simulink model "exDroopB_sim"  (R2014b)
settings: Solver=ode45  SolverMode=SingleTasking  StartTime=0.0  StopTime=15  MaxStep=0.0015  RelTol=1e-08
values from neighbouring files (symbols this model uses):
  bus1_vd = 2^0.5*1e3    (= 1414.21356237)    [ex3busPV.m]    (also in exLongLinePV.m = 141421.356237)
  Cbus_ext = 1e6*mpcC.bus(ssgen,BS)./(ws*baseV(ssgen).^2)    [exDroopA.m]    (also in exDroopB.m; exSyncGenPVinv.m)
  droop_Pref = 0.25*Pbase    (= 75000000)    [ex7busLongLine.m]    (also in exDroopA.m = mpc.gen(2:end,PG)*1e6; exDroopB.m = mpc.gen(:,PG)*1e6; exSyncGenPVinv.m = droop_Pref( [1:(synrp-1),(synrp+1):end]  ))
  droop_R = DROOP_R_GAIN_CNST./Prt    [ex7busLongLine.m]    (also in exDroopA.m; exDroopB.m)
  If_dc = 0.2*Prt./Ert    [ex14busSGandPV.m]    (also in ex7busLongLine.m = Prt./(60*Vf_dc); exDroopA.m = Prt./(60*Vf_dc); exDroopB.m = Prt./(60*Vf_dc); exSyncGenPVinv.m)
  J = J_GAIN_CNST*Prt/ws    [ex14busSGandPV.m]    (also in ex2busStability.m = 7.63943726841; ex7busLongLine.m = 2387.32414638; ex9busSG.m = J_GAIN_CNST*Pmax_gens/ws; exDroopA.m)
  Jtot = sum(J)    [exDroopB.m]
  Kd = KD_GAIN_CNST*J*ws    [ex14busSGandPV.m]    (also in ex2busStability.m = 24000; ex7busLongLine.m; ex9busSG.m; exDroopA.m)
  L0 = 0.1*Ld    [ex14busSGandPV.m]    (also in ex7busLongLine.m; exDroopA.m; exDroopB.m; exSyncGenPVinv.m)
  Laf = (2^0.5)*Ert./(ws*If_dc)    [ex14busSGandPV.m]    (also in ex7busLongLine.m; exDroopA.m; exDroopB.m; exSyncGenPVinv.m = (2^0.5)*5*Ert.^2./(ws*Prt))
  Lb2 = 2*Ld.*Lff - 3*Laf.^2    [ex14busSGandPV.m]    (also in ex7busLongLine.m; exDroopA.m; exDroopB.m; exSyncGenPVinv.m)
  Ld = 0.6*Lpu    [ex14busSGandPV.m]    (also in ex7busLongLine.m = 0.3*Lpu; exDroopA.m = 0.3*Lpu; exDroopB.m = 0.3*Lpu; exSyncGenPVinv.m)
  Lff = 2*Laf.^2./Ld    [ex14busSGandPV.m]    (also in ex7busLongLine.m; exDroopA.m; exDroopB.m; exSyncGenPVinv.m)
  Lq = Ld    [ex14busSGandPV.m]    (also in ex7busLongLine.m; exDroopA.m; exDroopB.m; exSyncGenPVinv.m)
  poles_2Jws = poles./(2*J*ws)    [ex14busSGandPV.m]    (also in ex2busStability.m = poles./(2*ws*J); ex7busLongLine.m; ex9busSG.m = poles./(2*ws*J); exDroopA.m)
  Ra = 0.05*Ert.^2./Prt    [ex14busSGandPV.m]    (also in ex7busLongLine.m = 0.01*Ert.^2./Prt; exDroopA.m = 0.01*Ert.^2./Prt; exDroopB.m = 0.01*Ert.^2./Prt; exSyncGenPVinv.m)
  Rf = Lff/1.2    [ex14busSGandPV.m]    (also in ex7busLongLine.m = Vf_dc./If_dc; exDroopA.m = Vf_dc./If_dc; exDroopB.m = Vf_dc./If_dc; exSyncGenPVinv.m)
  ssbus = [1; 2; 3; 6; 8]    [ex14busSGandPV.m]    (also in ex9busSG.m = [1 ; Genbus]; exDroopA.m = mpc.gen(:,GEN_BUS); exDroopB.m = mpc.gen(:,GEN_BUS); exLargeSysStability.m = mpc.gen(:,GEN_BUS))
  step_gen_num = 1    [exDroopB.m]
  step_size = 30e3    (= 30000)    [ex2busStability.m]    (also in exDroopB.m = 0)
  step_time = 9    [ex2busStability.m]    (also in ex3busPV.m = 0.05; exDroopB.m = 10; exLongLinePV.m = 1; syncMachVsSwing.m = 5)
  vcap_init_0 = 0*vppa    [exDroopA.m]    (also in exDroopB.m; exSyncGenPVinv.m)
  vcap_init_d = real(vppa)    [exDroopA.m]    (also in exDroopB.m; exSyncGenPVinv.m)
  vcap_init_q = imag(vppa)    [exDroopA.m]    (also in exDroopB.m; exSyncGenPVinv.m)
  Vf_dc = If_dc.*Rf    [ex14busSGandPV.m]    (also in ex7busLongLine.m = 500 * ones(size(Ert)); exDroopA.m = 500 * ones(size(Ert)); exDroopB.m = 500 * ones(size(Ert)); exSyncGenPVinv.m)
  ws = 2*pi*50    (= 314.159265359)    [ex14busSGandPV.m]    (also in ex2busStability.m; ex3busPV.m; ex7busLongLine.m; ex9busSG.m)
undefined symbols (not defined in the file or in its folder): Anet, Bnet, Cnet, Dnet, full
settings Model: Creator=COPEC  LastModifiedBy=Juri
settings OptimizationCC: BlockReduction=off  BooleanDataType=off
settings DebuggingCC: SaveWithParameterizedLinksMsg=none  UnderspecifiedInitializationDetection=Classic  MergeDetectMultiDrivingBlocksExec=none  SignalResolutionControl=TryResolveAllWithWarning  SolverPrmCheckMsg=none  FrameProcessingCompatibilityMsg=error
settings HardwareCC: TargetUnknown=on

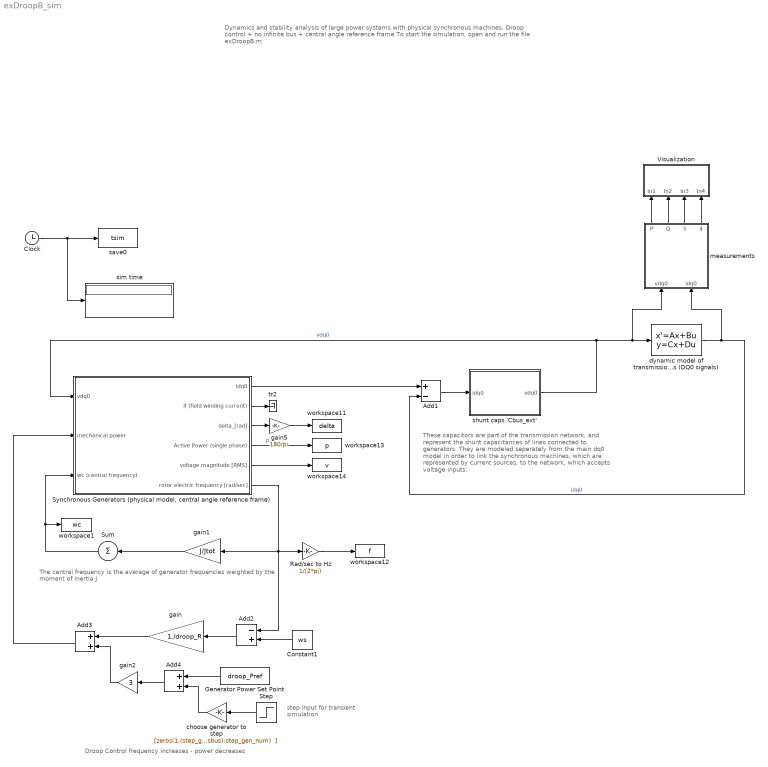
== system exDroopB_sim ==
  note: step input
      | for transient simulation
  note: Droop Control
      | frequency increases - power decreases
  note: Dynamics and stability analysis of large power systems
      | with physical synchronous machines.
      | Droop control + no infinite bus + central angle reference frame
      |
      | To start the simulation, open and run the file
      | exDroopB.m
  note: These capacitors are part of the transmission network, and represent the shunt capacitances of lines connected to generators. They are modeled seperately from the main dq0 model in order to link the synchronous machines, which are represented by current sources, to the network, which accepts voltage inputs.
  note: The central frequency is the average of generator
      | frequencies weighted by the moment of inertia J
  Add1 : Sum  Inputs=+-
  Add2 : Sum  Inputs=-+
  Add3 : Sum
  Add4 : Sum
  Clock : Clock
  Constant1 : Constant  Value=ws
  Generator Power Set Point : Constant  Value=droop_Pref
  Rad/sec to Hz : Gain  Gain=1/(2*pi)
  Step : Step  Time=step_time  After=step_size  SampleTime=0
  Sum : Sum  Inputs=+
  "Synchronous Generators (physical model, central angle reference frame)" : Subsystem
  Visualization : Subsystem
  choose generator to step : Gain  Gain="[zeros(1,(step_gen_num-1)) , 1 ,  zeros(1,length(ssbus)-step_gen_num)  ]"
  dynamic model of transmission network with integrated loads (DQ0 signals) : StateSpace  A=full(Anet)  B=full(Bnet)  C=full(Cnet)  D=full(Dnet)  X0=0
  gain : Gain  Gain=1./droop_R
  gain1 : Gain  Gain=J/Jtot
  gain2 : Gain  Gain=3
  gain5 : Gain  Gain=180/pi
  measurements : Subsystem
  save0 : ToWorkspace  VariableName=tsim  SampleTime=-1
  "shunt caps 'Cbus_ext' " : Subsystem
  sim time : Display
  tr2 : Terminator
  workspace1 : ToWorkspace  VariableName=wc  SampleTime=-1
  workspace11 : ToWorkspace  VariableName=delta  SampleTime=-1
  workspace12 : ToWorkspace  VariableName=f  SampleTime=-1
  workspace13 : ToWorkspace  VariableName=p  SampleTime=-1
  workspace14 : ToWorkspace  VariableName=v  SampleTime=-1
  wires:
  Clock/1 -> sim time/1, save0/1
  "Synchronous Generators (physical model, central angle reference frame)"/2(if (field winding current)) -> tr2/1
  "Synchronous Generators (physical model, central angle reference frame)"/3(delta_[rad]) -> gain5/1
  gain5/1 -> workspace11/1
  "Synchronous Generators (physical model, central angle reference frame)"/6(rotor electric frequency [rad/sec]) -> Add2/1, Rad/sec to Hz/1, gain1/1
  Rad/sec to Hz/1 -> workspace12/1
  "Synchronous Generators (physical model, central angle reference frame)"/4(Active Power (single phase)) -> workspace13/1  "p"
  "Synchronous Generators (physical model, central angle reference frame)"/5(voltage magnitude [RMS]) -> workspace14/1
  "Synchronous Generators (physical model, central angle reference frame)"/1(idq0) -> Add1/1
  Add1/1 -> "shunt caps 'Cbus_ext' "/1(idq0)
  "shunt caps 'Cbus_ext' "/1(vdq0) -> measurements/1(vdq0), dynamic model of transmission network with integrated loads (DQ0 signals)/1, "Synchronous Generators (physical model, central angle reference frame)"/1(vdq0)  "vdq0"
  dynamic model of transmission network with integrated loads (DQ0 signals)/1 -> measurements/2(idq0), Add1/2  "idq0"
  Constant1/1 -> Add2/2
  Add2/1 -> gain/1
  gain/1 -> Add3/1
  Add3/1 -> "Synchronous Generators (physical model, central angle reference frame)"/2(mechanical power)
  gain1/1 -> Sum/1
  Sum/1 -> workspace1/1, "Synchronous Generators (physical model, central angle reference frame)"/3(wc (central frequency))
  gain2/1 -> Add3/2
  choose generator to step/1 -> Add4/2
  Step/1 -> choose generator to step/1
  Add4/1 -> gain2/1
  Generator Power Set Point/1 -> Add4/1
  measurements/1(P) -> Visualization/1(In1)
  measurements/2(Q) -> Visualization/2(In2)
  measurements/3(Vm_RMS) -> Visualization/3(In3)
  measurements/4(Vph_deg) -> Visualization/4(In4)

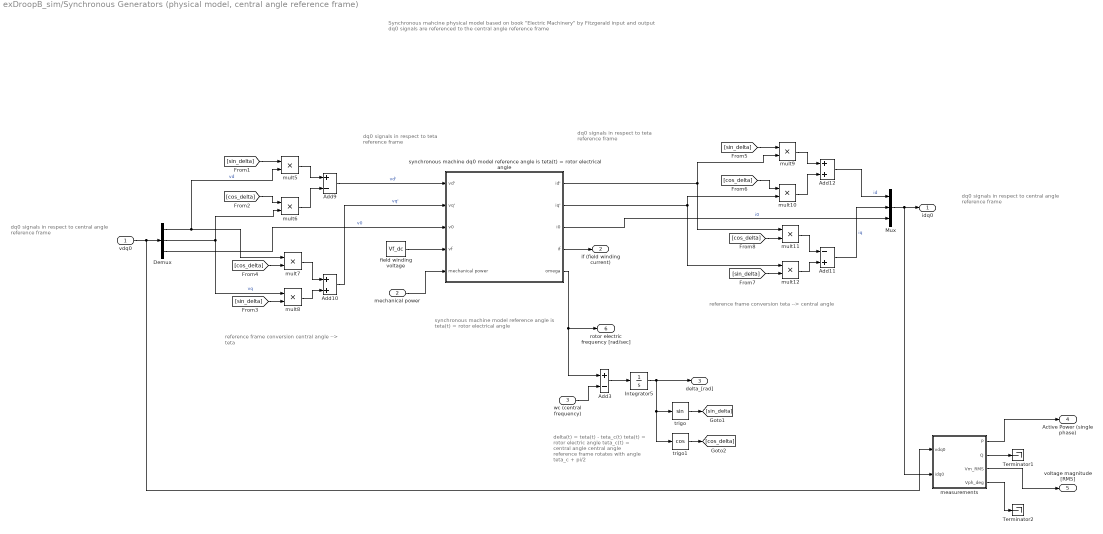
== system exDroopB_sim/Synchronous Generators (physical model, central angle reference frame) ==
  note: Synchronous mahcine physical model
      | based on book "Electric Machinery" by Fitzgerald
      |
      | input and output dq0 signals are referenced
      | to the central angle reference frame
  note: reference frame conversion central angle --> teta
  note: synchronous machine model
      | reference angle is
      | teta(t) = rotor electrical angle
  note: reference frame conversion teta --> central angle
  note: dq0 signals in respect to central angle reference frame
  note: dq0 signals in respect to teta reference frame
  note: dq0 signals in respect to teta reference frame
  note: delta(t) = teta(t) - teta_c(t)
      | teta(t) = rotor electric angle
      | teta_c(t) = central angle
      | central angle reference frame rotates with angle teta_c + pi/2
  note: dq0 signals in respect to central angle reference frame
  vdq0 : Inport
  mechanical power : Inport  Port=2
  wc (central frequency) : Inport  Port=3
  Add10 : Sum
  Add11 : Sum  Inputs=-+
  Add12 : Sum
  Add3 : Sum  Inputs=+-
  Add9 : Sum  Inputs=+-
  Demux : Demux  Outputs=3
  Integrator5 : Integrator
  Mux : Mux  Inputs=3
  Terminator1 : Terminator
  Terminator2 : Terminator
  field winding voltage : Constant  Value=Vf_dc
  measurements : Subsystem
  mult{5..12} (8 alike) : Product  Inputs=**
  synchronous machine dq0 model reference angle is teta(t) = rotor electrical angle : Subsystem
  trigo : Trigonometry
  trigo1 : Trigonometry  Operator=cos
  idq0 : Outport
  if (field winding current) : Outport  Port=2
  delta_[rad] : Outport  Port=3
  Active Power (single phase) : Outport  Port=4
  voltage magnitude [RMS] : Outport  Port=5
  rotor electric frequency [rad/sec] : Outport  Port=6
  wires:
  vdq0/1 -> measurements/1(vdq0), Demux/1
  Demux/1 -> mult5/2, mult7/1  "vd"
  Demux/2 -> mult6/2, mult8/1  "vq"
  mult5/1 -> Add9/1
  mult6/1 -> Add9/2
  [sin_delta] -> mult5/1
  [cos_delta] -> mult6/1
  mult7/1 -> Add10/1
  mult8/1 -> Add10/2
  [cos_delta] -> mult7/2
  [sin_delta] -> mult8/2
  mult9/1 -> Add12/1
  mult10/1 -> Add12/2
  [sin_delta] -> mult9/1
  [cos_delta] -> mult10/1
  mult11/1 -> Add11/1
  mult12/1 -> Add11/2
  [cos_delta] -> mult11/2
  [sin_delta] -> mult12/2
  Mux/1 -> measurements/2(idq0), idq0/1
  Add11/1 -> Mux/2  "iq"
  Add12/1 -> Mux/1  "id"
  synchronous machine dq0 model reference angle is teta(t) = rotor electrical angle/1(id') -> mult11/1, mult9/2
  synchronous machine dq0 model reference angle is teta(t) = rotor electrical angle/2(iq') -> mult12/1, mult10/2
  Add9/1 -> synchronous machine dq0 model reference angle is teta(t) = rotor electrical angle/1(vd')  "vd'"
  mechanical power/1 -> synchronous machine dq0 model reference angle is teta(t) = rotor electrical angle/5(mechanical power)
  Demux/3 -> synchronous machine dq0 model reference angle is teta(t) = rotor electrical angle/3(v0)  "v0"
  Add10/1 -> synchronous machine dq0 model reference angle is teta(t) = rotor electrical angle/2(vq')  "vq'"
  field winding voltage/1 -> synchronous machine dq0 model reference angle is teta(t) = rotor electrical angle/4(vf)
  synchronous machine dq0 model reference angle is teta(t) = rotor electrical angle/3(i0) -> Mux/3  "i0"
  synchronous machine dq0 model reference angle is teta(t) = rotor electrical angle/4(if) -> if (field winding current)/1
  trigo/1 -> [sin_delta]
  trigo1/1 -> [cos_delta]
  Add3/1 -> Integrator5/1
  synchronous machine dq0 model reference angle is teta(t) = rotor electrical angle/5(omega) -> Add3/1, rotor electric frequency [rad/sec]/1
  Integrator5/1 -> delta_[rad]/1, trigo1/1, trigo/1
  measurements/1(P) -> Active Power (single phase)/1
  measurements/2(Q) -> Terminator1/1
  measurements/3(Vm_RMS) -> voltage magnitude [RMS]/1
  measurements/4(Vph_deg) -> Terminator2/1
  wc (central frequency)/1 -> Add3/2

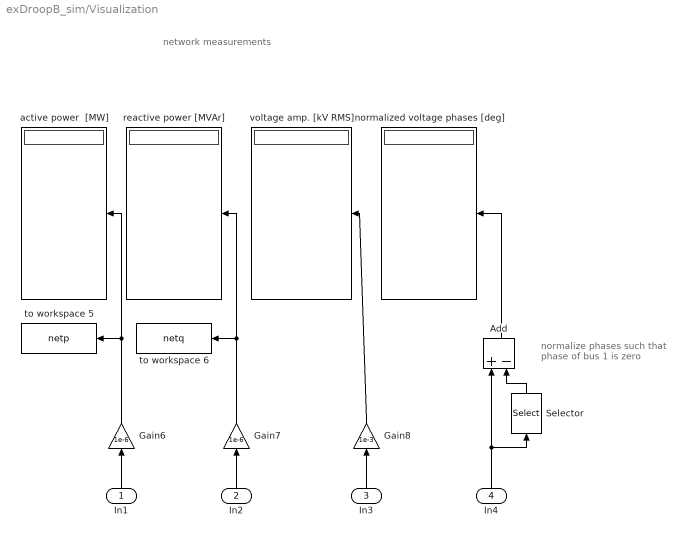
== system exDroopB_sim/Visualization ==
  note: normalize phases such that
      | phase of bus 1 is zero
  note: network measurements
  In1 : Inport
  In2 : Inport  Port=2
  In3 : Inport  Port=3
  In4 : Inport  Port=4
  Add : Sum  Inputs=+-
  Gain6 : Gain  Gain=1e-6
  Gain7 : Gain  Gain=1e-6
  Gain8 : Gain  Gain=1e-3
  Selector : Selector  InputPortWidth=length(ssbus)  IndexOptions=Index vector (dialog)  Indices=[1]  OutputSizes=1
  active power  [MW] : Display
  normalized voltage phases [deg] : Display
  reactive power [MVAr] : Display
  to workspace 5 : ToWorkspace  VariableName=netp  SampleTime=-1
  to workspace 6 : ToWorkspace  VariableName=netq  SampleTime=-1
  voltage amp. [kV RMS] : Display
  wires:
  Gain7/1 -> reactive power [MVAr]/1, to workspace 6/1
  Gain6/1 -> to workspace 5/1, active power  [MW]/1
  Gain8/1 -> voltage amp. [kV RMS]/1
  In2/1 -> Gain7/1
  In3/1 -> Gain8/1
  In4/1 -> Selector/1, Add/1
  In1/1 -> Gain6/1
  Selector/1 -> Add/2
  Add/1 -> normalized voltage phases [deg]/1

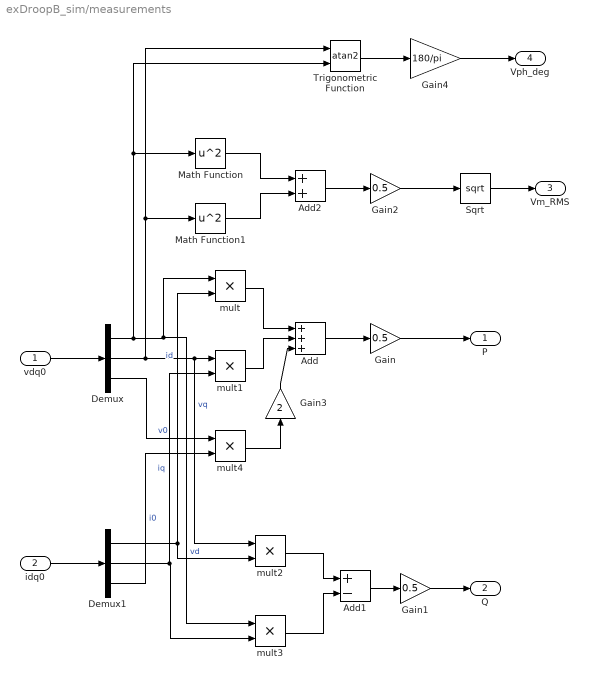
== system exDroopB_sim/measurements ==
  vdq0 : Inport
  idq0 : Inport  Port=2
  Add : Sum  Inputs=+++
  Add1 : Sum  Inputs=+-
  Add2 : Sum
  Demux : Demux  Outputs=3
  Demux1 : Demux  Outputs=3
  Gain : Gain  Gain=0.5
  Gain1 : Gain  Gain=0.5
  Gain2 : Gain  Gain=0.5
  Gain3 : Gain  Gain=2
  Gain4 : Gain  Gain=180/pi
  Math Function : Math  Operator=square  SaturateOnIntegerOverflow=on
  Math Function1 : Math  Operator=square  SaturateOnIntegerOverflow=on
  Sqrt : Sqrt  SaturateOnIntegerOverflow=on
  Trigonometric Function : Trigonometry  Operator=atan2
  mult{,1..4} (5 alike) : Product  Inputs=**
  P : Outport
  Q : Outport  Port=2
  Vm_RMS : Outport  Port=3
  Vph_deg : Outport  Port=4
  wires:
  idq0/1 -> Demux1/1
  vdq0/1 -> Demux/1
  Demux/1 -> Math Function/1, Trigonometric Function/2, mult3/1, mult/1  "vd"
  Demux/2 -> Trigonometric Function/1, Math Function1/1, mult2/1, mult1/1  "vq"
  Demux1/1 -> mult/2, mult2/2  "id"
  Demux1/2 -> mult3/2, mult1/2  "iq"
  Demux/3 -> mult4/1  "v0"
  Demux1/3 -> mult4/2  "i0"
  mult/1 -> Add/1
  mult1/1 -> Add/2
  Add/1 -> Gain/1
  mult2/1 -> Add1/1
  mult3/1 -> Add1/2
  Add1/1 -> Gain1/1
  Sqrt/1 -> Vm_RMS/1
  Math Function/1 -> Add2/1
  Math Function1/1 -> Add2/2
  Add2/1 -> Gain2/1
  Gain2/1 -> Sqrt/1
  Gain/1 -> P/1
  Gain1/1 -> Q/1
  mult4/1 -> Gain3/1
  Gain3/1 -> Add/3
  Trigonometric Function/1 -> Gain4/1
  Gain4/1 -> Vph_deg/1

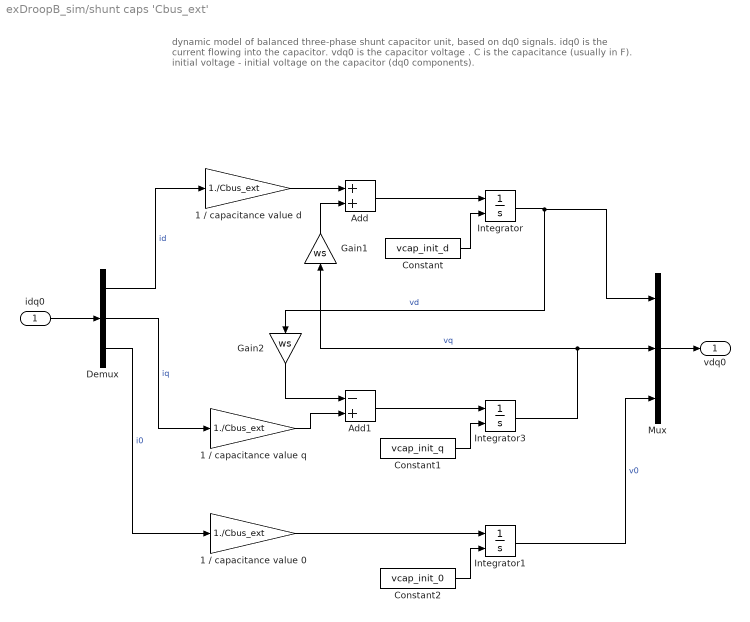
== system exDroopB_sim/shunt caps 'Cbus_ext'  ==
  note: dynamic model of balanced three-phase shunt capacitor unit, based on dq0 signals.
      | idq0 is the current flowing into the capacitor.
      | vdq0 is the capacitor voltage .
      | C is the capacitance (usually in F).
      | initial voltage - initial voltage on the capacitor (dq0 components).
  idq0 : Inport
  1 / capacitance value 0 : Gain  Gain=1./Cbus_ext
  1 / capacitance value d : Gain  Gain=1./Cbus_ext
  1 / capacitance value q : Gain  Gain=1./Cbus_ext
  Add : Sum
  Add1 : Sum  Inputs=-+
  Constant : Constant  Value=vcap_init_d
  Constant1 : Constant  Value=vcap_init_q
  Constant2 : Constant  Value=vcap_init_0
  Demux : Demux  Outputs=3
  Gain1 : Gain  Gain=ws
  Gain2 : Gain  Gain=ws
  Integrator : Integrator  InitialConditionSource=external  InitialCondition=bus1_vd
  Integrator1 : Integrator  InitialConditionSource=external  InitialCondition=bus1_vd
  Integrator3 : Integrator  InitialConditionSource=external  InitialCondition=bus1_vd
  Mux : Mux  Inputs=3
  vdq0 : Outport
  wires:
  Integrator1/1 -> Mux/3  "v0"
  Mux/1 -> vdq0/1
  Integrator/1 -> Gain2/1, Mux/1  "vd"
  Integrator3/1 -> Gain1/1, Mux/2  "vq"
  Add/1 -> Integrator/1
  Gain1/1 -> Add/2
  idq0/1 -> Demux/1
  1 / capacitance value d/1 -> Add/1
  Add1/1 -> Integrator3/1
  Gain2/1 -> Add1/1
  1 / capacitance value q/1 -> Add1/2
  1 / capacitance value 0/1 -> Integrator1/1
  Constant/1 -> Integrator/2
  Constant1/1 -> Integrator3/2
  Constant2/1 -> Integrator1/2
  Demux/1 -> 1 / capacitance value d/1  "id"
  Demux/2 -> 1 / capacitance value q/1  "iq"
  Demux/3 -> 1 / capacitance value 0/1  "i0"

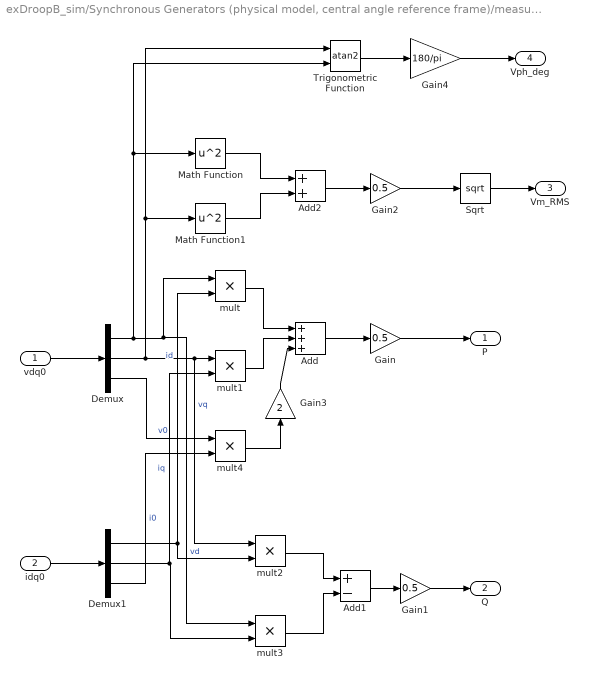
== system exDroopB_sim/Synchronous Generators (physical model, central angle reference frame)/measurements ==
  vdq0 : Inport
  idq0 : Inport  Port=2
  Add : Sum  Inputs=+++
  Add1 : Sum  Inputs=+-
  Add2 : Sum
  Demux : Demux  Outputs=3
  Demux1 : Demux  Outputs=3
  Gain : Gain  Gain=0.5
  Gain1 : Gain  Gain=0.5
  Gain2 : Gain  Gain=0.5
  Gain3 : Gain  Gain=2
  Gain4 : Gain  Gain=180/pi
  Math Function : Math  Operator=square  SaturateOnIntegerOverflow=on
  Math Function1 : Math  Operator=square  SaturateOnIntegerOverflow=on
  Sqrt : Sqrt  SaturateOnIntegerOverflow=on
  Trigonometric Function : Trigonometry  Operator=atan2
  mult{,1..4} (5 alike) : Product  Inputs=**
  P : Outport
  Q : Outport  Port=2
  Vm_RMS : Outport  Port=3
  Vph_deg : Outport  Port=4
  wires:
  idq0/1 -> Demux1/1
  vdq0/1 -> Demux/1
  Demux/1 -> Math Function/1, Trigonometric Function/2, mult3/1, mult/1  "vd"
  Demux/2 -> Trigonometric Function/1, Math Function1/1, mult2/1, mult1/1  "vq"
  Demux1/1 -> mult/2, mult2/2  "id"
  Demux1/2 -> mult3/2, mult1/2  "iq"
  Demux/3 -> mult4/1  "v0"
  Demux1/3 -> mult4/2  "i0"
  mult/1 -> Add/1
  mult1/1 -> Add/2
  Add/1 -> Gain/1
  mult2/1 -> Add1/1
  mult3/1 -> Add1/2
  Add1/1 -> Gain1/1
  Sqrt/1 -> Vm_RMS/1
  Math Function/1 -> Add2/1
  Math Function1/1 -> Add2/2
  Add2/1 -> Gain2/1
  Gain2/1 -> Sqrt/1
  Gain/1 -> P/1
  Gain1/1 -> Q/1
  mult4/1 -> Gain3/1
  Gain3/1 -> Add/3
  Trigonometric Function/1 -> Gain4/1
  Gain4/1 -> Vph_deg/1

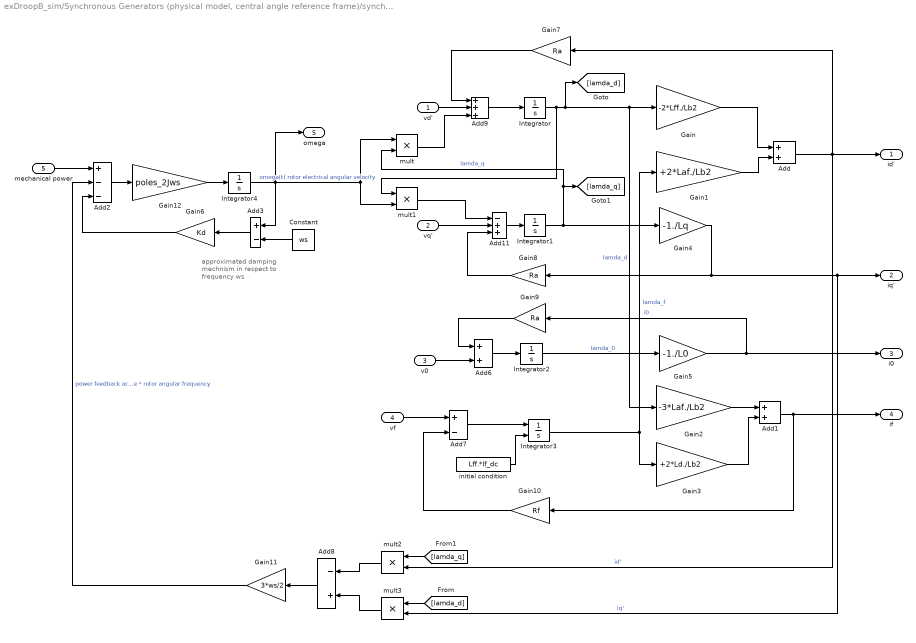
== system exDroopB_sim/Synchronous Generators (physical model, central angle reference frame)/synchronous machine dq0 model reference angle is teta(t) = rotor electrical angle ==
  note: approximated damping
      | mechnism in respect to
      | frequency ws
  vd' : Inport
  vq' : Inport  Port=2
  v0 : Inport  Port=3
  vf : Inport  Port=4
  mechanical power : Inport  Port=5
  Add : Sum
  Add1 : Sum
  Add11 : Sum  Inputs=-++
  Add2 : Sum  Inputs=+--
  Add3 : Sum  Inputs=+-
  Add6 : Sum
  Add7 : Sum  Inputs=+-
  Add8 : Sum  Inputs=-+
  Add9 : Sum  Inputs=+++
  Constant : Constant  Value=ws
  Gain : Gain  Gain=-2*Lff./Lb2
  Gain1 : Gain  Gain=+2*Laf./Lb2
  Gain10 : Gain  Gain=Rf
  Gain11 : Gain  Gain=3*ws/2
  Gain12 : Gain  Gain=poles_2Jws
  Gain2 : Gain  Gain=-3*Laf./Lb2
  Gain3 : Gain  Gain=+2*Ld./Lb2
  Gain4 : Gain  Gain=-1./Lq
  Gain5 : Gain  Gain=-1./L0
  Gain6 : Gain  Gain=Kd
  Gain7 : Gain  Gain=Ra
  Gain8 : Gain  Gain=Ra
  Gain9 : Gain  Gain=Ra
  Integrator : Integrator
  Integrator1 : Integrator
  Integrator2 : Integrator
  Integrator3 : Integrator  InitialConditionSource=external  InitialCondition=Lff(1)*If_dc(1)
  Integrator4 : Integrator  InitialCondition=ws
  initial condition : Constant  Value=Lff.*If_dc
  mult{,1..3} (4 alike) : Product  Inputs=**
  id' : Outport
  iq' : Outport  Port=2
  i0 : Outport  Port=3
  if : Outport  Port=4
  omega : Outport  Port=5
  wires:
  Gain1/1 -> Add/2
  Add6/1 -> Integrator2/1
  mechanical power/1 -> Add2/1
  Gain6/1 -> Add2/3
  Integrator/1 -> mult1/1, Gain2/1, Gain/1, [lamda_d]  "lamda_d"
  Gain5/1 -> i0/1, Gain9/1  "i0"
  Integrator1/1 -> Gain4/1, [lamda_q], mult/2  "lamda_q"
  Integrator2/1 -> Gain5/1  "lamda_0"
  Integrator3/1 -> Gain1/1, Gain3/1  "lamda_f"
  Add1/1 -> if/1, Gain10/1
  Gain4/1 -> iq'/1, mult3/2, Gain8/1  "iq'"
  Add/1 -> mult2/2, id'/1, Gain7/1  "id'"
  Gain/1 -> Add/1
  vf/1 -> Add7/1
  Add7/1 -> Integrator3/1
  Gain9/1 -> Add6/1
  Add8/1 -> Gain11/1
  Gain11/1 -> Add2/2  "power feedback acting to slow the rotor = Torque * rotor angular frequency"
  Gain8/1 -> Add11/3
  mult/1 -> Add9/3
  mult1/1 -> Add11/1
  Add9/1 -> Integrator/1
  vd'/1 -> Add9/2
  Gain3/1 -> Add1/2
  Gain2/1 -> Add1/1
  Gain10/1 -> Add7/2
  Add11/1 -> Integrator1/1
  Gain7/1 -> Add9/1
  mult3/1 -> Add8/2
  mult2/1 -> Add8/1
  v0/1 -> Add6/2
  Add3/1 -> Gain6/1
  Constant/1 -> Add3/2
  vq'/1 -> Add11/2
  [lamda_q] -> mult2/1
  [lamda_d] -> mult3/1
  Integrator4/1 -> omega/1, Add3/1, mult1/2, mult/1  "omega(t) rotor electrical angular velocity"
  Add2/1 -> Gain12/1
  Gain12/1 -> Integrator4/1
  initial condition/1 -> Integrator3/2
